simulink model "myLKS2"  (R2013b)
settings: Solver=ode45  StartTime=0.0  StopTime=10.0  RelTol=1e-3
model workspace (MAT data in the model file):
  Cf = 72653
  Cr = 121449
  Fy_Angle = [-20; -16; -14; -12; -10; -9.5; -9; -8.5; -8; -7.5; -7; -6.5; -6; -5.5; -5; -4.5; -4; -3.5; -3; -2.5; -2; -1.5; -1; -0.5; 0; 0.5; 1; 1.5; 2; 2.5; 3; 3.5; 4; 4.5; 5; 5.5; 6; 6.5; 7; 7.5; 8; 8.5; 9; 9.5; 10; 12; 14; 16; 18; 20]
  Fy_Data = [-1523.64 -1531.91 -1546.58 -1574.53 -1631.62 -1653.27 -1678.67 -1707.8 -1740.18 -1775.12 -1810.95 -1845.3 ... (250 elements, 50x5)]
  Fy_W = [1725 3500 6100 6950 9005]
  GearRatio = 17.25
  Izz = 3746
  lf = 1.17
  lr = 1.77
  m = 1820
values from neighbouring files (symbols this model uses):
  psi0 = 0 * (pi/180)    (= 0)    [MainLKS.m]
  X0 = 0    [MainLKS.m]
  Y0 = 1    [MainLKS.m]
undefined symbols (not defined in the file or in its folder): A, B, K, L, sigbuilder_block
settings Model: Creator=IVDL  LastModifiedBy=edward
settings DataIOCC: SignalLoggingSaveFormat=ModelDataLogs
settings DebuggingCC: UnderspecifiedInitializationDetection=Simplified  MultiTaskDSMMsg=warning  MultiTaskCondExecSysMsg=none  StrictBusMsg=None
settings RTWCC: IncludeERTFirstTime=on
settings GRTTargetCC: CodeReplacementLibrary=None  CPPClassGenCompliant=on

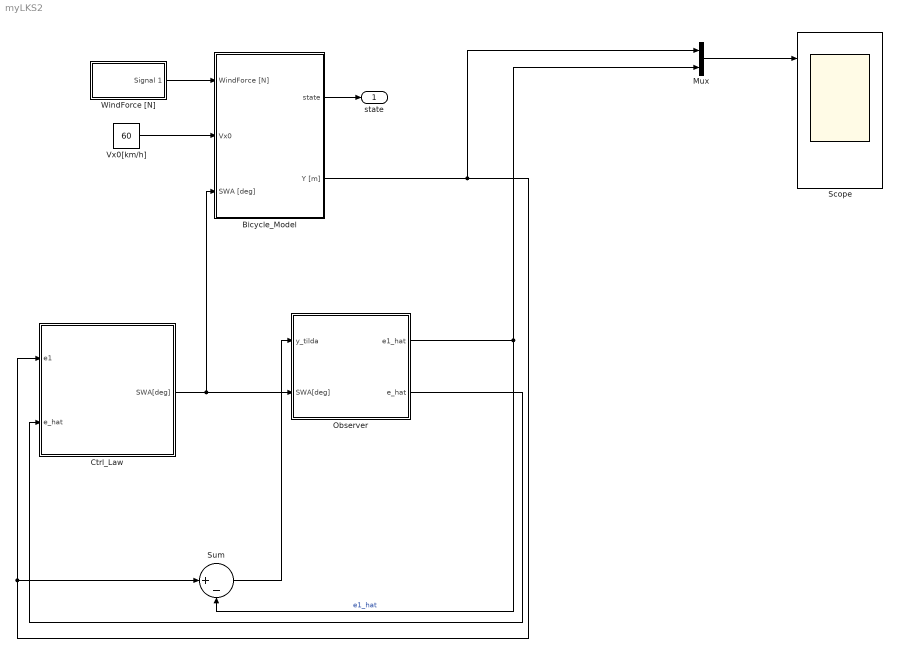
== system myLKS2 ==
  Bicycle_Model : Subsystem
  Ctrl_Law : Subsystem
  Mux : Mux  Inputs=2
  Observer : Subsystem
  Scope : Scope  NumInputPorts=3
      settings: YMin=-5~-5~-5  YMax=5~5~5
  Sum : Sum  Inputs=|+-
  Vx0[km/h] : Constant  Value=60
  WindForce [N] : Subsystem  Tag=STV Subsys  LoadFcn=sigbuilder_block('load');  StartFcn=sigbuilder_block('start');  StopFcn=sigbuilder_block('stop');  ClipboardFcn=sigbuilder_block('clipboard');  mask(Sigbuilder block){}
      mask help: Simulink:masks:SigbuilderBlock_MD
      mask init:
      | if ~strcmp(get_param(bdroot(gcbh),'SimulationStatus'),'stopped') tuvar = sigbuilder_block('maskInit'); end
      settings: CopyFcn=sigbuilder_block('copy');  DeleteFcn=sigbuilder_block('delete');  ModelCloseFcn=sigbuilder_block('modelClose');  PreSaveFcn=sigbuilder_block('preSave');  PauseFcn=sigbuilder_block('pause');  ContinueFcn=sigbuilder_block('continue');  NameChangeFcn=sigbuilder_block('namechange');  OpenFcn=sigbuilder_block('open',[437.25 199.5 550.5 399.75 ]);  CloseFcn=sigbuilder_block('close');
      mask Display: plot(0, 0, 100, 100,[2, 2, 32, 32, 2], [68, 8, 8, 68, 68],[32, 2], [38, 38], [32, 19, 2],[53, 60, 44], [32, 17, 17, 2],[16, 16, 31, 31]);txt = getActiveGroup(gcbh);text(2, 100, txt,'verticalAlignment', 'top');
  state : Outport
  wires:
  WindForce [N]/1(Signal 1) -> Bicycle_Model/1(WindForce [N])
  Sum/1 -> Observer/1(y_tilda)
  Observer/2(e_hat) -> Ctrl_Law/2(e_hat)
  Ctrl_Law/1(SWA[deg]) -> Bicycle_Model/3(SWA [deg]), Observer/2(SWA[deg])
  Observer/1(e1_hat) -> Sum/2, Mux/2  "e1_hat"
  Vx0[km/h]/1 -> Bicycle_Model/2(Vx0)
  Bicycle_Model/1(state) -> state/1
  Bicycle_Model/2(Y [m]) -> Mux/1, Ctrl_Law/1(e1), Sum/1
  Mux/1 -> Scope/1

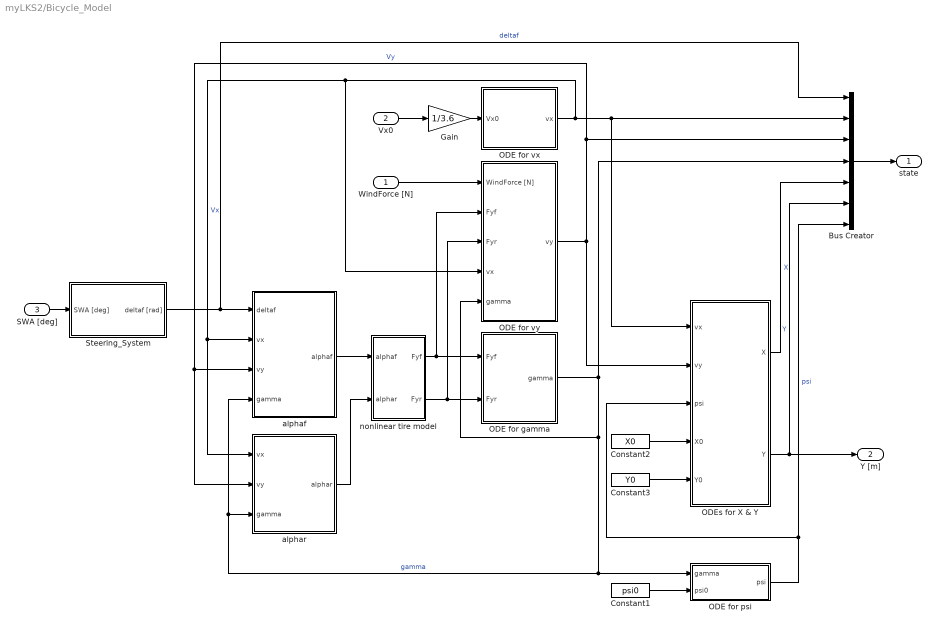
== system myLKS2/Bicycle_Model ==
  WindForce [N] : Inport
  Vx0 : Inport  Port=2
  SWA [deg] : Inport  Port=3
  Bus Creator : BusCreator  Inputs=7
  Constant1 : Constant  Value=psi0
  Constant2 : Constant  Value=X0
  Constant3 : Constant  Value=Y0
  Gain : Gain  Gain=1/3.6
  ODE for gamma : Subsystem
  ODE for psi : Subsystem
  ODE for vx : Subsystem
  ODE for vy : Subsystem
  ODEs for X & Y : Subsystem
  Steering_System : Subsystem
  alphaf : Subsystem
  alphar : Subsystem
  nonlinear tire model : Subsystem
  state : Outport
  Y [m] : Outport  Port=2
  wires:
  alphaf/1(alphaf) -> nonlinear tire model/1(alphaf)
  alphar/1(alphar) -> nonlinear tire model/2(alphar)
  nonlinear tire model/1(Fyf) -> ODE for gamma/1(Fyf), ODE for vy/2(Fyf)
  nonlinear tire model/2(Fyr) -> ODE for gamma/2(Fyr), ODE for vy/3(Fyr)
  ODE for gamma/1(gamma) -> Bus Creator/4, ODE for vy/5(gamma), alphar/3(gamma), alphaf/4(gamma), ODE for psi/1(gamma)  "gamma"
  ODE for vy/1(vy) -> alphaf/3(vy), alphar/2(vy), Bus Creator/3, ODEs for X & Y/2(vy)  "Vy"
  Bus Creator/1 -> state/1
  ODE for vx/1(vx) -> Bus Creator/2, ODEs for X & Y/1(vx), alphaf/2(vx), alphar/1(vx), ODE for vy/4(vx)  "Vx"
  Vx0/1 -> Gain/1
  Constant1/1 -> ODE for psi/2(psi0)
  Gain/1 -> ODE for vx/1(Vx0)
  SWA [deg]/1 -> Steering_System/1(SWA [deg])
  Constant2/1 -> ODEs for X & Y/4(X0)
  Constant3/1 -> ODEs for X & Y/5(Y0)
  ODE for psi/1(psi) -> Bus Creator/7, ODEs for X & Y/3(psi)  "psi"
  ODEs for X & Y/1(X) -> Bus Creator/5  "X"
  ODEs for X & Y/2(Y) -> Bus Creator/6, Y [m]/1  "Y"
  Steering_System/1(deltaf [rad]) -> alphaf/1(deltaf), Bus Creator/1  "deltaf"
  WindForce [N]/1 -> ODE for vy/1(WindForce [N])

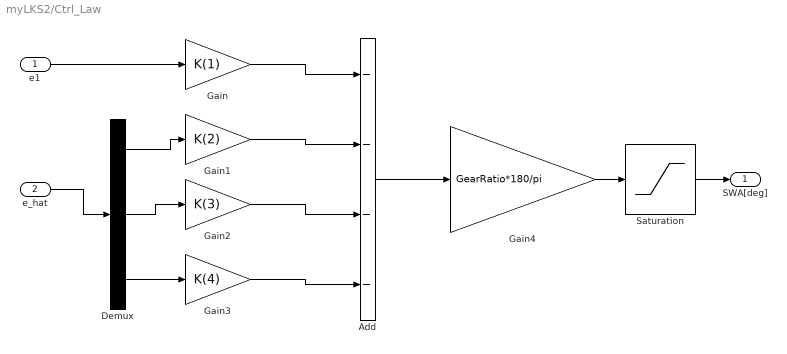
== system myLKS2/Ctrl_Law ==
  e1 : Inport
  e_hat : Inport  Port=2
  Add : Sum  Inputs=----
  Demux : Demux  Outputs=3
  Gain : Gain  Gain=K(1)
  Gain1 : Gain  Gain=K(2)
  Gain2 : Gain  Gain=K(3)
  Gain3 : Gain  Gain=K(4)
  Gain4 : Gain  Gain=GearRatio*180/pi
  Saturation : Saturate  UpperLimit=450  LowerLimit=-450
  SWA[deg] : Outport
  wires:
  Gain1/1 -> Add/2
  Gain/1 -> Add/1
  Gain4/1 -> Saturation/1
  Gain3/1 -> Add/4
  Saturation/1 -> SWA[deg]/1
  Gain2/1 -> Add/3
  Demux/2 -> Gain2/1
  Demux/3 -> Gain3/1
  e_hat/1 -> Demux/1
  Demux/1 -> Gain1/1
  e1/1 -> Gain/1
  Add/1 -> Gain4/1

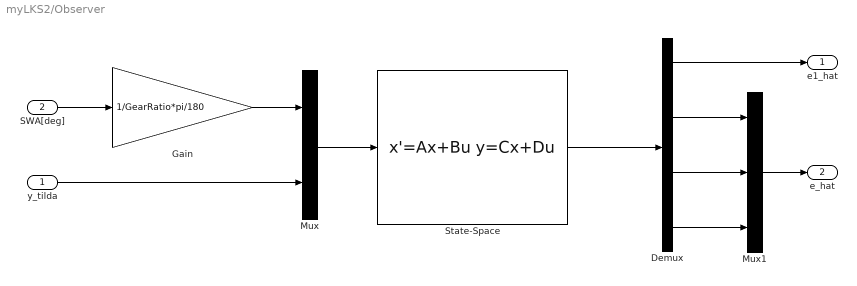
== system myLKS2/Observer ==
  y_tilda : Inport
  SWA[deg] : Inport  Port=2
  Demux : Demux
  Gain : Gain  Gain=1/GearRatio*pi/180
  Mux : Mux  Inputs=2
  Mux1 : Mux  Inputs=3
  State-Space : StateSpace  A=A  B=[B L']  C=diag([1 1 1 1])  D=zeros(4,2)  X0=0  ContinuousStateAttributes={'e1','e1_dot','e2','e2_dot'}
  e1_hat : Outport
  e_hat : Outport  Port=2
  wires:
  SWA[deg]/1 -> Gain/1
  Gain/1 -> Mux/1
  y_tilda/1 -> Mux/2
  State-Space/1 -> Demux/1
  Demux/3 -> Mux1/2
  Mux1/1 -> e_hat/1
  Demux/1 -> e1_hat/1
  Mux/1 -> State-Space/1
  Demux/2 -> Mux1/1
  Demux/4 -> Mux1/3

== system myLKS2/WindForce [N] ==
  Demux : Demux  Tag=STV Demux  Outputs=1
  FromWs : FromWorkspace  Tag=STV FromWs  VariableName=tuvar  SampleTime=0
      SigBuilderData=|
      | common.afterFinalStr = 'Extrapolate'
      | common.sampleTime = 0
      | dataSet.timeRange = [0 10]
      | dataSet.name = 'Group 1'
      | sbobj.Groups.Name = 'Group 1'
      | sbobj.Groups.Signals.Name = 'Signal 1'
      | sbobj.Groups.Signals.XData = [0 1 1 1.1 1.1 10]
      | sbobj.Groups.Signals.YData = [0 0 30 30 0 0]
  Signal 1 : Outport  Tag=STV Outport
  wires:
  Demux/1 -> Signal 1/1
  FromWs/1 -> Demux/1

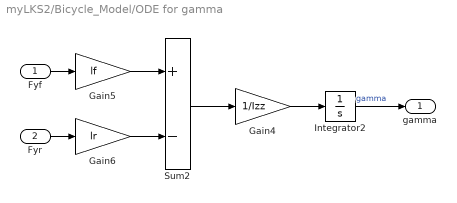
== system myLKS2/Bicycle_Model/ODE for gamma ==
  Fyf : Inport
  Fyr : Inport  Port=2
  Gain4 : Gain  Gain=1/Izz
  Gain5 : Gain  Gain=lf
  Gain6 : Gain  Gain=lr
  Integrator2 : Integrator
  Sum2 : Sum  Inputs=+-
  gamma : Outport
  wires:
  Sum2/1 -> Gain4/1
  Gain4/1 -> Integrator2/1
  Gain5/1 -> Sum2/1
  Gain6/1 -> Sum2/2
  Fyf/1 -> Gain5/1
  Integrator2/1 -> gamma/1  "gamma"
  Fyr/1 -> Gain6/1

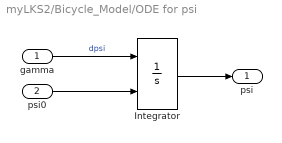
== system myLKS2/Bicycle_Model/ODE for psi ==
  gamma : Inport
  psi0 : Inport  Port=2
  Integrator : Integrator  InitialConditionSource=external
  psi : Outport
  wires:
  gamma/1 -> Integrator/1  "dpsi"
  Integrator/1 -> psi/1
  psi0/1 -> Integrator/2

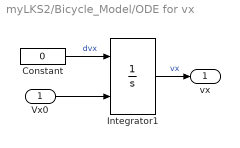
== system myLKS2/Bicycle_Model/ODE for vx ==
  Vx0 : Inport
  Constant : Constant  Value=0
  Integrator1 : Integrator  InitialConditionSource=external  InitialCondition=80/3.6
  vx : Outport
  wires:
  Constant/1 -> Integrator1/1  "dvx"
  Integrator1/1 -> vx/1  "vx"
  Vx0/1 -> Integrator1/2

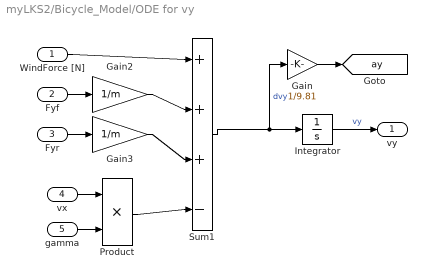
== system myLKS2/Bicycle_Model/ODE for vy ==
  WindForce [N] : Inport
  Fyf : Inport  Port=2
  Fyr : Inport  Port=3
  vx : Inport  Port=4
  gamma : Inport  Port=5
  Gain : Gain  Gain=1/9.81
  Gain2 : Gain  Gain=1/m
  Gain3 : Gain  Gain=1/m
  Integrator : Integrator
  Product : Product  RndMeth=Zero
  Sum1 : Sum  Inputs=+++|-
  vy : Outport
  tag scope: ay=global
  wires:
  Gain2/1 -> Sum1/2
  Gain3/1 -> Sum1/3
  Sum1/1 -> Gain/1, Integrator/1  "dvy"
  Product/1 -> Sum1/4
  Fyf/1 -> Gain2/1
  Fyr/1 -> Gain3/1
  Integrator/1 -> vy/1  "vy"
  vx/1 -> Product/1
  gamma/1 -> Product/2
  Gain/1 -> [ay]
  WindForce [N]/1 -> Sum1/1

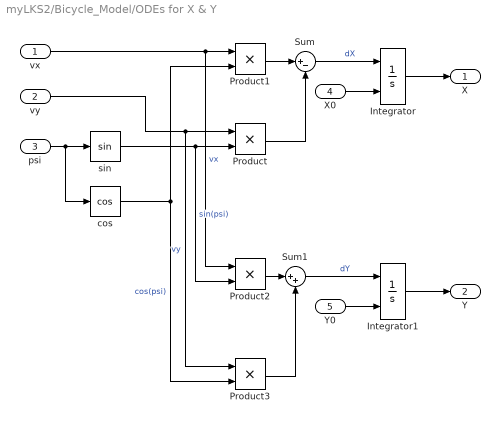
== system myLKS2/Bicycle_Model/ODEs for X & Y ==
  vx : Inport
  vy : Inport  Port=2
  psi : Inport  Port=3
  X0 : Inport  Port=4
  Y0 : Inport  Port=5
  Integrator : Integrator  InitialConditionSource=external  InitialCondition=42.14
  Integrator1 : Integrator  InitialConditionSource=external  InitialCondition=-0.3743
  Product{,1..3} (4 alike) : Product  RndMeth=Zero
  Sum : Sum  Inputs=|+-
  Sum1 : Sum  Inputs=|++
  cos : Trigonometry  Operator=cos
  sin : Trigonometry
  X : Outport
  Y : Outport  Port=2
  wires:
  psi/1 -> sin/1, cos/1
  sin/1 -> Product/2, Product2/2  "sin(psi)"
  vy/1 -> Product/1, Product3/1  "vy"
  vx/1 -> Product1/1, Product2/1  "vx"
  cos/1 -> Product1/2, Product3/2  "cos(psi)"
  Product1/1 -> Sum/1
  Product/1 -> Sum/2
  Sum/1 -> Integrator/1  "dX"
  Product2/1 -> Sum1/1
  Product3/1 -> Sum1/2
  Sum1/1 -> Integrator1/1  "dY"
  Integrator/1 -> X/1
  Integrator1/1 -> Y/1
  X0/1 -> Integrator/2
  Y0/1 -> Integrator1/2

== system myLKS2/Bicycle_Model/Steering_System ==
  SWA [deg] : Inport
  Gain : Gain  Gain=1/GearRatio
  Gain5 : Gain  Gain=pi/180
  deltaf [rad] : Outport
  wires:
  Gain/1 -> Gain5/1
  Gain5/1 -> deltaf [rad]/1
  SWA [deg]/1 -> Gain/1

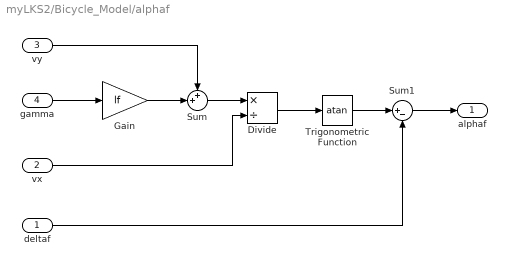
== system myLKS2/Bicycle_Model/alphaf ==
  deltaf : Inport
  vx : Inport  Port=2
  vy : Inport  Port=3
  gamma : Inport  Port=4
  Divide : Product  Inputs=*/
  Gain : Gain  Gain=lf
  Sum : Sum  Inputs=++|
  Sum1 : Sum  Inputs=|+-
  Trigonometric Function : Trigonometry  Operator=atan
  alphaf : Outport
  wires:
  gamma/1 -> Gain/1
  vy/1 -> Sum/1
  Gain/1 -> Sum/2
  Sum/1 -> Divide/1
  vx/1 -> Divide/2
  Divide/1 -> Trigonometric Function/1
  Trigonometric Function/1 -> Sum1/1
  deltaf/1 -> Sum1/2
  Sum1/1 -> alphaf/1

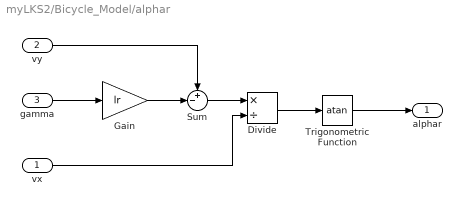
== system myLKS2/Bicycle_Model/alphar ==
  vx : Inport
  vy : Inport  Port=2
  gamma : Inport  Port=3
  Divide : Product  Inputs=*/
  Gain : Gain  Gain=lr
  Sum : Sum  Inputs=+-|
  Trigonometric Function : Trigonometry  Operator=atan
  alphar : Outport
  wires:
  Trigonometric Function/1 -> alphar/1
  Divide/1 -> Trigonometric Function/1
  vx/1 -> Divide/2
  Sum/1 -> Divide/1
  Gain/1 -> Sum/2
  vy/1 -> Sum/1
  gamma/1 -> Gain/1

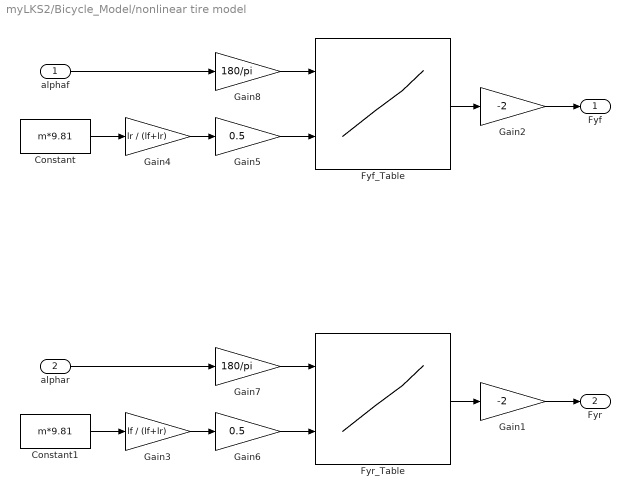
== system myLKS2/Bicycle_Model/nonlinear tire model ==
  alphaf : Inport
  alphar : Inport  Port=2
  Constant : Constant  Value=m*9.81
  Constant1 : Constant  Value=m*9.81
  Fyf_Table : Lookup2D  RowIndex=Fy_Angle  ColumnIndex=Fy_W  Table=Fy_Data  LookUpMeth=Interpolation-Use End Values  SaturateOnIntegerOverflow=on
  Fyr_Table : Lookup2D  RowIndex=Fy_Angle  ColumnIndex=Fy_W  Table=Fy_Data  LookUpMeth=Interpolation-Use End Values  SaturateOnIntegerOverflow=on
  Gain1 : Gain  Gain=-2
  Gain2 : Gain  Gain=-2
  Gain3 : Gain  Gain=lf / (lf+lr)
  Gain4 : Gain  Gain=lr / (lf+lr)
  Gain5 : Gain  Gain=0.5
  Gain6 : Gain  Gain=0.5
  Gain7 : Gain  Gain=180/pi
  Gain8 : Gain  Gain=180/pi
  Fyf : Outport
  Fyr : Outport  Port=2
  wires:
  alphaf/1 -> Gain8/1
  Constant/1 -> Gain4/1
  Gain4/1 -> Gain5/1
  Gain5/1 -> Fyf_Table/2
  Fyf_Table/1 -> Gain2/1
  Gain2/1 -> Fyf/1
  Gain8/1 -> Fyf_Table/1
  alphar/1 -> Gain7/1
  Gain3/1 -> Gain6/1
  Gain6/1 -> Fyr_Table/2
  Fyr_Table/1 -> Gain1/1
  Gain7/1 -> Fyr_Table/1
  Constant1/1 -> Gain3/1
  Gain1/1 -> Fyr/1
